simulink model "MIL4L3_SW6_V1_20220211"  (R2018b)
settings: Solver=FixedStepAuto  StartTime=0.0  StopTime=inf  FixedStep=0.001  RelTol=1e-3
PreLoadFcn:
  | A0_MILtest;
undefined symbols (not defined in the file or in its folder): Clb_ICADirect_LaneDisp_StateFive, Clb_ICADirect_LaneDisp_StateFour, Clb_ICADirect_LaneDisp_StateOne, Clb_ICADirect_LaneDisp_StateThree, Clb_ICADirect_LaneDisp_StateTwo, Clb_ICADirect_LaneDisp_StateZero, Clb_ICADirect_LaneDispSW, Clb_ICADirect_TrnLghtsCom_Switch, Clb_ICADirect_TrnLghtsCom_Value, Clb_ICADirect_TrnLghtsCrtl_Inhb, IMAP_Clb_ACU_Driver_Belt, IMAP_Clb_ACU_Driver_Belt_Over, IMAP_Clb_ACU_Passenger_Belt, IMAP_Clb_ACU_Passenger_Belt_Over, IMAP_Clb_ACU_RearLeft_Belt, IMAP_Clb_ACU_RearLeft_Belt_Over, IMAP_Clb_ACU_RearMiddle_Belt, IMAP_Clb_ACU_RearMiddle_Belt_Over, IMAP_Clb_ACU_RearRight_Belt, IMAP_Clb_ACU_RearRight_Belt_Over, IMAP_Clb_AEB_Switch, IMAP_Clb_AEB_Switch_Over, IMAP_Clb_ALC_TLC_Mode, IMAP_Clb_ALC_TLC_Mode_Over, IMAP_Clb_BCM_Battery_Voltage, IMAP_Clb_BCM_Battery_Voltage_Over, IMAP_Clb_BCM_BrakeLamp_State, IMAP_Clb_BCM_BrakeLamp_State_Over, IMAP_Clb_BCM_CHMSL_Status, IMAP_Clb_BCM_CHMSL_Status_Over, IMAP_Clb_BCM_Door_Lock_State, IMAP_Clb_BCM_Door_Lock_State_Over, IMAP_Clb_BCM_FrontWiper_State, IMAP_Clb_BCM_FrontWiper_State_Over, IMAP_Clb_BCM_FrontWiper_Switch, IMAP_Clb_BCM_FrontWiper_Switch_Over, IMAP_Clb_BCM_HazardLamp, IMAP_Clb_BCM_HazardLamp_Over, IMAP_Clb_BCM_HazardLamp_Switch, IMAP_Clb_BCM_HazardLamp_Switch_Over, IMAP_Clb_BCM_HighBeam_State, IMAP_Clb_BCM_HighBeam_State_Over, IMAP_Clb_BCM_Ignition_State, IMAP_Clb_BCM_Ignition_State_Over, IMAP_Clb_BCM_IHBC_Enabled, IMAP_Clb_BCM_IHBC_Enabled_Over, IMAP_Clb_BCM_Left_Light, IMAP_Clb_BCM_Left_Light_Over, IMAP_Clb_BCM_LeftTurn_Switch, IMAP_Clb_BCM_LeftTurn_Switch_Over, IMAP_Clb_BCM_LF_Door_State, IMAP_Clb_BCM_LF_Door_State_Over, IMAP_Clb_BCM_LowBeam_State, IMAP_Clb_BCM_LowBeam_State_Over, IMAP_Clb_BCM_LR_Door_State, IMAP_Clb_BCM_LR_Door_State_Over, IMAP_Clb_BCM_RF_Door_State, IMAP_Clb_BCM_RF_Door_State_Over, IMAP_Clb_BCM_Right_Light, IMAP_Clb_BCM_Right_Light_Over ... (+547)
libraries: CarMaker4SL x2153, simulink x292, dspstat3 x3, canmsglib x2, simulink_extras x1
(part 2 of 52)

== system MIL4L3_SW6_V1_20220211/CarMaker/VehicleControl/OMAP ==
  note: 转向灯控制命令
  note: ACC时距间隔显示
  note: 飞轮扭矩激活请求
  note: 驾驶员设置ACC巡航速度
  note: ACC文字提示
  note: AEB FCW报警请求信号
  note: AEB &FCW Fault 指示灯
  note: AEB OFF指示灯
  note: AEB 文字提示
  note: ACC轮端请求扭矩
  note: ACC状态
  note: 减速度设置
  note: 减速度控制请求
  note: 预建压请求
  note: 减速度类型
  note: AEB状态
  note: 刹车请求(AEB/IBA/ACC共用)
  note: 振动报警请求
  note: 脱手报警
  note: LDW 报警状态
  note: LDW Only 状态指示
  note: 摄像头发出的LKA功能模式
  note: LKA状态指示
  note: LKA功能开启状态
  note: ELK功能指示灯
  note: LKA状态
  note: LKA请求的目标转角
  note: ESA状态
  note: ICA_弹出文字提醒
  note: ICA_状态灯
  note: 多车道模式指示
  note: 提醒驾驶员打转向灯
  note: ESA扭矩请求
  note: ESA请求
  note: 0 No Request
      | 1 左转向灯亮
      | 2 右转向灯亮
      | 3 左右双闪
  note: 1 左
      | 2 右
  Bus Selector2 : BusSelector  Commented=on  OutputSignals=AEBSve_d_Prefill_request,AEBSve_d_functionFARCState,AEBSve_g_DecSetpoint,AEBSve_d_MDDdecRequest,AEBSve_d_MDDdecType,AEBSve_d_ESCDriverOff,AEBSve_d_ESCHoldReq,AEBSve_d_HapticAlarm,AEBSve_d_Braking_progress,AEBSve_d_AEBStatus,AEBSve_d_FCWStatus,AEBSve_d_AEBSwitchStatus,AEBSve_d_AEBFaultStatus,AEBSve_d_AEBAlertReq,AEBSve_d_AEBTips,AEBSve_d_SignalTStamp,AEBSve_d_JABS_AlertSign,AEBSve_d_JABS_SwitchStatus,AEBSve_d_JABS_FltStatus,AEBSve_d_JABS_AlertReq,AEBSve_d_JABS_HapticAlarm,AEBSve_d_JABS_Tips
  Bus Selector3 : BusSelector  OutputSignals=LKASve_y_Vehicle_Lane_Display,LKASve_y_LDW_Status_Display,LKASve_y_LKA_Status_Display,LKASve_y_LDW_Flag,LKASve_y_Hands_Off_Warning,LKASve_y_LKA_Action_Indication,LKASve_y_HMI_Popup_Status,LKASve_y_EPS_State_Control,LKASve_g_LKA_SWA_Control,LKASve_g_EPS_Factor_Control,LKASve_y_EPS_LKA_Control,LKASve_y_LKATorqueReq,LKASve_g_LKATorqueReq_Value
  Bus Selector4 : BusSelector  OutputSignals=JABSve_d_DbPrefillReq,JABSve_d_DbFunFARCSta,JABSve_g_DbDecSetpoint,JABSve_d_DbMDDdecRequest,JABSve_d_DbMDDdecType,JABSve_d_DbHapticAlarm,JABSve_d_DbBraking_progress,JABSve_d_DbSignalTStamp,JABSve_d_DbJACWStatus,JABSve_d_DbSwitchStatus,JABSve_d_DbFltStatus,JABSve_d_DbAlertReq,JABSve_d_DbTips,JABSve_d_DbESCDriveOff,JABSve_d_DbESCHoldReq
  Bus Selector6 : BusSelector  Commented=on  OutputSignals=ELKSve_y_state_ELK_function,ELKSve_y_ELK_HapticAlarmReq,ELKSve_y_Hands_Off_Warning,ELKSve_y_ELK_Action_Indication,ELKSve_y_HMI_Popup_Status,ELKSve_y_EPS_State_Control,ELKSve_g_ELK_SWA_Control,ELKSve_g_EPS_Factor_Control,ELKSve_y_EPS_ELK_Control,ELKSve_y_ELK_VehicleLaneDisp,ELKSve_y_ELK_ELKSts,ELKSve_y_SignalTStamp,ELKSve_y_LKATorqueReq,ELKSve_g_LKATorqueReq_Value
  Bus Selector7 : BusSelector  OutputSignals=IMAPve_d_EPS_LKA_State,IMAPve_g_ESC_LonAcc,IMAPva_d_obj_id,IMAPva_g_obj_pos_x,IMAPve_d_ESC_Veh_Standstill,IMAPve_g_L0_C0,IMAPve_g_L0_C1,IMAPve_g_L0_C2,IMAPve_g_L0_C3,IMAPve_g_R0_C0,IMAPve_g_R0_C1,IMAPve_g_R0_C2,IMAPve_g_R0_C3,IMAPve_d_APA_AutoPark_WorkSt
  Bus Selector8 : BusSelector  Commented=on  OutputSignals=ESASve_y_ESA_State,ESASve_g_ESA_SWA_CMD,ESASve_g_EPS_Factor_Control,ESASve_y_ESA_FaultSt,ESASve_y_ESARequest,ESASve_y_ESATorqueReq,ESASve_y_LKAActivation
  Bus Selector9 : BusSelector  Commented=on  OutputSignals=IMAPve_d_L0_Q,IMAPve_d_R0_Q
  Bus Selector : BusSelector  OutputSignals=FDMMve_d_JaFcnConf,FDMMve_d_AebFcnConf,FDMMve_d_EsaFcnConf,FDMMve_d_ElkFcnConf,FDMMve_d_LkaFcnConf,FDMMve_d_IcaFcnConf,FDMMve_d_AccFcnConf,FDMMve_d_EwFcnConf,FDMMve_g_Adas2Fapa,FDMMve_d_SignalTStamp
  Bus Selector1 : BusSelector  Commented=on  OutputSignals=ACCSve_d_ACC_State,ACCSve_g_ACC_TqReq,ACCSve_d_ACC_TqFlag,ACCSve_g_ACC_DecReq,ACCSve_d_ACC_DecFlag,ACCSve_d_CIPV_ID,ACCSve_d_ACCActive_Signal,ACCSve_d_ACC_go_request,ACCSve_d_VelocitySet,ACCSve_d_HeadWaySet,ACCSve_d_SignalTStamp,ACCSve_d_ACC_ICA_Flag,ACCSve_d_ACC_ESCDriverOff,ACCSve_d_ACC_ESCHoldReq,ACCSve_d_ACC_EPBReq,ACCSve_d_ACCMessagePrompt,ACCSve_d_ACC_ISLCState,ACCSve_d_ACC_ISLCDriverRemind
  Bus Selector5 : BusSelector  Commented=on  OutputSignals=ICABve_d_SignalTStamp,ICABva_d_ICAB2HMI,ICABve_g_SteerAngleCmd,ICABve_d_ICAMode,ICABve_d_ICAState,ICABve_d_LKATorqueReq,ICABve_g_LKATorqueReq_Value
  Data Type  Conversion{,1..2,4..9} (9 alike) : DataTypeConversion
  Data Type Conversion{,2..12,175,180,253..262,264..270,302..304} (34 alike) : DataTypeConversion
  Data Type Conversion1 : DataTypeConversion  Commented=on
  Define CM Dict : CarMaker4SL/Define CM Dict  xname=User.IO.In.ADAS_ACCState  xmono=on  xtype=Int  xdvaplace=None  xnstates=0  xfirststate=0  xinitial=0
  Define CM Dict1 : CarMaker4SL/Define CM Dict  xname=User.IO.In.ADAS_LDWWarningSt  xmono=off  xtype=Double4  xdvaplace=VC  xnstates=0  xfirststate=0  xinitial=0
  Define CM Dict11 : CarMaker4SL/Define CM Dict  xname=User.IO.In.ADAS_LKAAngleReq  xunit=degree  xmono=off  xtype=Double  xdvaplace=IO_In  xnstates=0  xfirststate=0  xinitial=0
  Define CM Dict12 : CarMaker4SL/Define CM Dict  xname=User.IO.In.ADAS_ICAStatusIcon  xmono=off  xtype=Double4  xdvaplace=IO_In  xnstates=0  xfirststate=0  xinitial=0
  Define CM Dict14 : CarMaker4SL/Define CM Dict  xname=User.IO.In.ADAS_ACCTorqueReq  xmono=off  xtype=Double  xdvaplace=None  xnstates=0  xfirststate=0  xinitial=0
  Define CM Dict15 : CarMaker4SL/Define CM Dict  xname=User.IO.In.ADAS_ESCDriveOff  xmono=off  xtype=Double4  xdvaplace=VC  xnstates=0  xfirststate=0  xinitial=0
  Define CM Dict16 : CarMaker4SL/Define CM Dict  xname=User.IO.In.ADAS_ACCSetSpeed  xunit=km/h  xmono=off  xtype=Double  xdvaplace=None  xnstates=0  xfirststate=0  xinitial=0
  Define CM Dict17 : CarMaker4SL/Define CM Dict  xname=User.IO.In.ADAS_ACCHeadwayDisplay  xmono=off  xtype=Double  xdvaplace=None  xnstates=0  xfirststate=0  xinitial=0
  Define CM Dict18 : CarMaker4SL/Define CM Dict  xname=User.IO.In.ADAS_DecelerationSetpoint  xunit=m/s^2  xmono=off  xtype=Double  xdvaplace=None  xnstates=0  xfirststate=0  xinitial=0
  Define CM Dict19 : CarMaker4SL/Define CM Dict  xname=User.IO.In.ADAS_LKAState  xmono=off  xtype=Double  xdvaplace=IO_In  xnstates=0  xfirststate=0  xinitial=0
  Define CM Dict2 : CarMaker4SL/Define CM Dict  Commented=on  xname=User.IO.In.ICA_Mode  xmono=off  xtype=Double4  xdvaplace=VC  xnstates=0  xfirststate=0  xinitial=0
  Define CM Dict20 : CarMaker4SL/Define CM Dict  xname=User.IO.In.ADAS_ISAMessageDisp  xmono=off  xtype=Double4  xdvaplace=IO_In  xnstates=0  xfirststate=0  xinitial=0
  Define CM Dict21 : CarMaker4SL/Define CM Dict  xname=User.IO.In.ADAS_PowerWheelTorqueActiveReq  xmono=off  xtype=Double4  xdvaplace=IO_In  xnstates=0  xfirststate=0  xinitial=0
  Define CM Dict22 : CarMaker4SL/Define CM Dict  xname=User.IO.In.ADAS_ESCHoldReq  xmono=off  xtype=Double4  xdvaplace=VC  xnstates=0  xfirststate=0  xinitial=0
  Define CM Dict23 : CarMaker4SL/Define CM Dict  xname=User.IO.In.ADAS_AEBState  xmono=off  xtype=Double4  xdvaplace=VC  xnstates=0  xfirststate=0  xinitial=0
  Define CM Dict24 : CarMaker4SL/Define CM Dict  xname=User.IO.In.ADAS_AEBAlertReq  xmono=off  xtype=Double4  xdvaplace=VC  xnstates=0  xfirststate=0  xinitial=0
  Define CM Dict25 : CarMaker4SL/Define CM Dict  xname=User.IO.In.ADAS_HapticAlarmRequest  xmono=off  xtype=Double4  xdvaplace=VC  xnstates=0  xfirststate=0  xinitial=0
  Define CM Dict28 : CarMaker4SL/Define CM Dict  xname=User.IO.In.ADAS_DecelerationType  xmono=off  xtype=Double4  xdvaplace=VC  xnstates=0  xfirststate=0  xinitial=0
  Define CM Dict29 : CarMaker4SL/Define CM Dict  xname=User.IO.In.ADAS_DecelerationControlReq  xmono=off  xtype=Double4  xdvaplace=VC  xnstates=0  xfirststate=0  xinitial=0
  Define CM Dict3 : CarMaker4SL/Define CM Dict  xname=User.IO.In.ADAS_ACCMessagePrompt  xmono=off  xtype=Double4  xdvaplace=IO_In  xnstates=0  xfirststate=0  xinitial=0
  Define CM Dict30 : CarMaker4SL/Define CM Dict  xname=User.IO.In.ADAS_AEBFaultStatus  xmono=off  xtype=Double4  xdvaplace=VC  xnstates=0  xfirststate=0  xinitial=0
  Define CM Dict31 : CarMaker4SL/Define CM Dict  xname=User.IO.In.ADAS_AEBSwitchStatus  xmono=off  xtype=Double4  xdvaplace=VC  xnstates=0  xfirststate=0  xinitial=0
  Define CM Dict32 : CarMaker4SL/Define CM Dict  xname=User.IO.In.ADAS_AEBMessageDisp  xmono=off  xtype=Double4  xdvaplace=VC  xnstates=0  xfirststate=0  xinitial=0
  Define CM Dict33 : CarMaker4SL/Define CM Dict  xname=User.IO.In.ADAS_Handoffwarning  xmono=off  xtype=Double4  xdvaplace=VC  xnstates=0  xfirststate=0  xinitial=0
  Define CM Dict34 : CarMaker4SL/Define CM Dict  xname=User.IO.In.ADAS_PrefillRequest  xmono=off  xtype=Double4  xdvaplace=VC  xnstates=0  xfirststate=0  xinitial=0
  Define CM Dict35 : CarMaker4SL/Define CM Dict  xname=User.IO.In.ADAS_ESAFault  xmono=off  xtype=Double4  xdvaplace=IO_In  xnstates=0  xfirststate=0  xinitial=0
  Define CM Dict36 : CarMaker4SL/Define CM Dict  xname=User.IO.In.ADAS_JAFault  xmono=off  xtype=Double4  xdvaplace=IO_In  xnstates=0  xfirststate=0  xinitial=0
  Define CM Dict37 : CarMaker4SL/Define CM Dict  xname=User.IO.In.ADAS_TurnLightsCommand  xmono=off  xtype=Double4  xdvaplace=IO_In  xnstates=0  xfirststate=0  xinitial=0
  Define CM Dict38 : CarMaker4SL/Define CM Dict  xname=User.IO.In.ADAS_ISL_CDriverRemind  xmono=off  xtype=Double  xdvaplace=IO_In  xnstates=0  xfirststate=0  xinitial=0
  Define CM Dict39 : CarMaker4SL/Define CM Dict  xname=User.IO.In.ADAS_LKAStatusDisplay  xmono=off  xtype=Double4  xdvaplace=VC  xnstates=0  xfirststate=0  xinitial=0
  Define CM Dict4 : CarMaker4SL/Define CM Dict  xname=User.IO.In.ADAS_LKASwitchState  xmono=off  xtype=Double4  xdvaplace=VC  xnstates=0  xfirststate=0  xinitial=0
  Define CM Dict40 : CarMaker4SL/Define CM Dict  xname=User.IO.In.ADAS_LKAMode  xmono=off  xtype=Double4  xdvaplace=VC  xnstates=0  xfirststate=0  xinitial=0
  Define CM Dict41 : CarMaker4SL/Define CM Dict  xname=User.IO.In.ADAS_VehicleLaneDisplay  xmono=off  xtype=Double4  xdvaplace=VC  xnstates=0  xfirststate=0  xinitial=0
  Define CM Dict42 : CarMaker4SL/Define CM Dict  xname=User.IO.In.ADAS_HWAActionSts  xmono=off  xtype=Double4  xdvaplace=IO_In  xnstates=0  xfirststate=0  xinitial=0
  Define CM Dict44 : CarMaker4SL/Define CM Dict  xname=User.IO.In.ADAS_LDWStatusDisplay  xmono=off  xtype=Double4  xdvaplace=VC  xnstates=0  xfirststate=0  xinitial=0
  Define CM Dict48 : CarMaker4SL/Define CM Dict  xname=User.IO.In.ADAS_HWAMode  xmono=off  xtype=Double4  xdvaplace=IO_In  xnstates=0  xfirststate=0  xinitial=0
  Define CM Dict5 : CarMaker4SL/Define CM Dict  xname=User.IO.In.ADAS_ELKSts  xmono=off  xtype=Double4  xdvaplace=VC  xnstates=0  xfirststate=0  xinitial=0
  Define CM Dict50 : CarMaker4SL/Define CM Dict  xname=User.IO.In.ADAS_HWATurnOnIndicator  xmono=off  xtype=Double4  xdvaplace=IO_In  xnstates=0  xfirststate=0  xinitial=0
  Define CM Dict51 : CarMaker4SL/Define CM Dict  xname=User.IO.In.ADAS_ESATorqueReq  xmono=off  xtype=Double  xdvaplace=IO_In  xnstates=0  xfirststate=0  xinitial=0
  Define CM Dict52 : CarMaker4SL/Define CM Dict  xname=User.IO.In.ADAS_ESARequest  xmono=off  xtype=Double  xdvaplace=IO_In  xnstates=0  xfirststate=0  xinitial=0
  Define CM Dict6 : CarMaker4SL/Define CM Dict  xname=User.IO.In.ADAS_ESAState  xmono=off  xtype=Double  xdvaplace=IO_In  xnstates=0  xfirststate=0  xinitial=0
  Define CM Dict7 : CarMaker4SL/Define CM Dict  xname=User.IO.In.ADAS_ISLCState  xmono=off  xtype=Double  xdvaplace=IO_In  xnstates=0  xfirststate=0  xinitial=0
  Define CM Dict8 : CarMaker4SL/Define CM Dict  xname=User.IO.In.ADAS_ACCHeadwayIcon  xmono=off  xtype=Double  xdvaplace=None  xnstates=0  xfirststate=0  xinitial=0
  Define CM Dict9 : CarMaker4SL/Define CM Dict  xname=User.IO.In.ADAS_BrakeRequest  xmono=off  xtype=Double4  xdvaplace=VC  xnstates=0  xfirststate=0  xinitial=0
  Delay : Delay  DelayLength=1
  From : From  Commented=on  GotoTag=ESA_output  TagVisibility=global
  From19 : From  Commented=on  GotoTag=ACC_output  TagVisibility=global
  From33 : From  Commented=on  GotoTag=AEB_output  TagVisibility=global
  From37 : From  Commented=on  GotoTag=ELK_output  TagVisibility=global
  From38 : From  Commented=on  GotoTag=ICAB_output  TagVisibility=global
  Goto7 : Goto  Commented=on  GotoTag=Decel_Request  TagVisibility=global
  Manual Switch : ManualSwitch
  OMAP1 : Subsystem  TreatAsAtomicUnit=on  SystemSampleTime=0.01
  Write CM Dict : CarMaker4SL/Write CM Dict  xname=User.IO.In.ADAS_LDWWarningSt  xsync=off
  Write CM Dict1 : CarMaker4SL/Write CM Dict  xname=User.IO.In.ADAS_BrakeRequest  xsync=off
  Write CM Dict10 : CarMaker4SL/Write CM Dict  xname=User.IO.In.ADAS_ISAMessageDisp  xsync=off
  Write CM Dict11 : CarMaker4SL/Write CM Dict  xname=User.IO.In.ADAS_LKAState  xsync=off
  Write CM Dict12 : CarMaker4SL/Write CM Dict  xname=User.IO.In.ADAS_PowerWheelTorqueActiveReq  xsync=off
  Write CM Dict13 : CarMaker4SL/Write CM Dict  xname=User.IO.In.ADAS_ACCMessagePrompt  xsync=off
  Write CM Dict14 : CarMaker4SL/Write CM Dict  xname=User.IO.In.ADAS_AEBState  xsync=off
  Write CM Dict15 : CarMaker4SL/Write CM Dict  xname=User.IO.In.ADAS_AEBAlertReq  xsync=off
  Write CM Dict16 : CarMaker4SL/Write CM Dict  xname=User.IO.In.ADAS_HapticAlarmRequest  xsync=off
  Write CM Dict19 : CarMaker4SL/Write CM Dict  xname=User.IO.In.ADAS_DecelerationType  xsync=off
  Write CM Dict2 : CarMaker4SL/Write CM Dict  xname=User.IO.In.ADAS_ACCState  xsync=off
  Write CM Dict20 : CarMaker4SL/Write CM Dict  xname=User.IO.In.ADAS_DecelerationControlReq  xsync=off
  Write CM Dict21 : CarMaker4SL/Write CM Dict  xname=User.IO.In.ADAS_AEBFaultStatus  xsync=off
  Write CM Dict22 : CarMaker4SL/Write CM Dict  xname=User.IO.In.ADAS_AEBSwitchStatus  xsync=off
  Write CM Dict23 : CarMaker4SL/Write CM Dict  xname=User.IO.In.ADAS_AEBMessageDisp  xsync=off
  Write CM Dict24 : CarMaker4SL/Write CM Dict  xname=User.IO.In.ADAS_Handoffwarning  xsync=off
  Write CM Dict25 : CarMaker4SL/Write CM Dict  xname=User.IO.In.ADAS_PrefillRequest  xsync=off
  Write CM Dict26 : CarMaker4SL/Write CM Dict  Commented=on  xname=User.IO.In.ICA_Mode  xsync=off
  Write CM Dict27 : CarMaker4SL/Write CM Dict  xname=User.IO.In.ADAS_LKAStatusDisplay  xsync=off
  Write CM Dict28 : CarMaker4SL/Write CM Dict  xname=User.IO.In.ADAS_LKAMode  xsync=off
  Write CM Dict29 : CarMaker4SL/Write CM Dict  xname=User.IO.In.ADAS_LDWStatusDisplay  xsync=off
  Write CM Dict30 : CarMaker4SL/Write CM Dict  xname=User.IO.In.ADAS_HWAMode  xsync=off
  Write CM Dict31 : CarMaker4SL/Write CM Dict  xname=User.IO.In.ADAS_LKASwitchState  xsync=off
  Write CM Dict32 : CarMaker4SL/Write CM Dict  xname=User.IO.In.ADAS_ELKSts  xsync=off
  Write CM Dict33 : CarMaker4SL/Write CM Dict  xname=User.IO.In.ADAS_ESAState  xsync=off
  Write CM Dict34 : CarMaker4SL/Write CM Dict  xname=User.IO.In.ADAS_HWATurnOnIndicator  xsync=off
  Write CM Dict35 : CarMaker4SL/Write CM Dict  xname=User.IO.In.ADAS_ESATorqueReq  xsync=off
  Write CM Dict36 : CarMaker4SL/Write CM Dict  xname=User.IO.In.ADAS_ESARequest  xsync=off
  Write CM Dict37 : CarMaker4SL/Write CM Dict  xname=User.IO.In.ADAS_ISLCState  xsync=off
  Write CM Dict38 : CarMaker4SL/Write CM Dict  xname=User.IO.In.ADAS_ACCHeadwayIcon  xsync=off
  Write CM Dict39 : CarMaker4SL/Write CM Dict  xname=User.IO.In.ADAS_ESCDriveOff  xsync=off
  Write CM Dict4 : CarMaker4SL/Write CM Dict  xname=User.IO.In.ADAS_ACCTorqueReq  xsync=off
  Write CM Dict40 : CarMaker4SL/Write CM Dict  xname=User.IO.In.ADAS_ESCHoldReq  xsync=off
  Write CM Dict41 : CarMaker4SL/Write CM Dict  xname=User.IO.In.ADAS_ESAFault  xsync=off
  Write CM Dict42 : CarMaker4SL/Write CM Dict  xname=User.IO.In.ADAS_JAFault  xsync=off
  Write CM Dict43 : CarMaker4SL/Write CM Dict  xname=User.IO.In.ADAS_TurnLightsCommand  xsync=off
  Write CM Dict44 : CarMaker4SL/Write CM Dict  xname=User.IO.In.ADAS_ISL_CDriverRemind  xsync=off
  Write CM Dict45 : CarMaker4SL/Write CM Dict  xname=User.IO.In.ADAS_VehicleLaneDisplay  xsync=off
  Write CM Dict46 : CarMaker4SL/Write CM Dict  xname=User.IO.In.ADAS_HWAActionSts  xsync=off
  Write CM Dict5 : CarMaker4SL/Write CM Dict  xname=User.IO.In.ADAS_ACCSetSpeed  xsync=off
  Write CM Dict6 : CarMaker4SL/Write CM Dict  xname=User.IO.In.ADAS_ACCHeadwayDisplay  xsync=off
  Write CM Dict7 : CarMaker4SL/Write CM Dict  xname=User.IO.In.ADAS_DecelerationSetpoint  xsync=off
  Write CM Dict8 : CarMaker4SL/Write CM Dict  xname=User.IO.In.ADAS_LKAAngleReq  xsync=off
  Write CM Dict9 : CarMaker4SL/Write CM Dict  xname=User.IO.In.ADAS_ICAStatusIcon  xsync=off
  tag scope: ACCTqReq=global, ADAS_AEBAlertReq=global, ADAS_DecelerationSet=global, ADAS_TorqueActivReq=global, MDD_Decelerationcontrol_request=global, MDD_deceleration_type=global
  wires:
  [JA_output] -> Bus Selector4/1
  From33/1 -> Bus Selector2/1
  From19/1 -> Bus Selector1/1
  [LKA_output] -> Bus Selector3/1
  From38/1 -> Bus Selector5/1
  [FDMM_output] -> Bus Selector/1
  Data Type Conversion302/1 -> Write CM Dict27/1
  From37/1 -> Bus Selector6/1
  Data Type Conversion260/1 -> Write CM Dict13/1
  Data Type Conversion264/1 -> Write CM Dict19/1
  Data Type Conversion1/1 -> Write CM Dict26/1
  Data Type Conversion304/1 -> Write CM Dict29/1
  Data Type Conversion268/1 -> Write CM Dict23/1
  Data Type  Conversion1/1 -> Write CM Dict10/1
  Data Type Conversion259/1 -> Write CM Dict12/1
  Data Type Conversion267/1 -> Write CM Dict22/1
  Data Type Conversion253/1 -> Write CM Dict5/1
  Data Type Conversion258/1 -> Write CM Dict11/1
  Data Type Conversion303/1 -> Write CM Dict28/1
  Data Type Conversion/1 -> Write CM Dict2/1
  Data Type Conversion175/1 -> Write CM Dict/1
  OMAP1/10(OMAPve_y_ADAS_AEBAlertReq) -> Data Type Conversion261/1, [ADAS_AEBAlertReq]
  Manual Switch/1 -> Data Type  Conversion/1
  Data Type Conversion257/1 -> Write CM Dict8/1
  Data Type  Conversion/1 -> Write CM Dict9/1
  Data Type Conversion262/1 -> Write CM Dict16/1
  Data Type Conversion270/1 -> Write CM Dict25/1
  Data Type Conversion266/1 -> Write CM Dict21/1
  Bus Selector5/4 -> OMAP1/96(ICABve_d_ICAMode), Data Type Conversion1/1  "<ICABve_d_ICAMode>"
  Data Type Conversion269/1 -> Write CM Dict24/1
  Data Type Conversion265/1 -> Write CM Dict20/1
  Data Type Conversion254/1 -> Write CM Dict6/1
  Data Type Conversion256/1 -> Write CM Dict4/1
  Data Type  Conversion2/1 -> Write CM Dict14/1
  Data Type Conversion255/1 -> Write CM Dict7/1
  Data Type Conversion180/1 -> Write CM Dict1/1
  Data Type Conversion2/1 -> Write CM Dict31/1
  Data Type Conversion3/1 -> Write CM Dict32/1
  Data Type Conversion4/1 -> Write CM Dict33/1
  Bus Selector2/1 -> OMAP1/29(AEBSve_d_Prefill_request)  "<AEBSve_d_Prefill_request>"
  Bus Selector2/2 -> OMAP1/30(AEBSve_d_functionFARCState)  "<AEBSve_d_functionFARCState>"
  Bus Selector2/3 -> OMAP1/31(AEBSve_g_DecSetpoint)  "<AEBSve_g_DecSetpoint>"
  Bus Selector2/4 -> OMAP1/32(AEBSve_d_MDDdecRequest)  "<AEBSve_d_MDDdecRequest>"
  Bus Selector2/5 -> OMAP1/33(AEBSve_d_MDDdecType)  "<AEBSve_d_MDDdecType>"
  Bus Selector2/6 -> OMAP1/34(AEBSve_d_ESCDriveOff)  "<AEBSve_d_ESCDriverOff>"
  Bus Selector2/7 -> OMAP1/35(AEBSve_d_ESCHoldReq)  "<AEBSve_d_ESCHoldReq>"
  Bus Selector2/8 -> OMAP1/36(AEBSve_d_HapticAlarm)  "<AEBSve_d_HapticAlarm>"
  Bus Selector2/9 -> OMAP1/37(AEBSve_d_Braking_progress)  "<AEBSve_d_Braking_progress>"
  Bus Selector2/10 -> OMAP1/38(AEBSve_d_AEBStatus)  "<AEBSve_d_AEBStatus>"
  Bus Selector2/11 -> OMAP1/39(AEBSve_d_FCWStatus)  "<AEBSve_d_FCWStatus>"
  Bus Selector2/12 -> OMAP1/40(AEBSve_d_AEBSwitchStatus)  "<AEBSve_d_AEBSwitchStatus>"
  Bus Selector2/13 -> OMAP1/41(AEBSve_d_AEBFaultStatus)  "<AEBSve_d_AEBFaultStatus>"
  Bus Selector2/14 -> OMAP1/42(AEBSve_d_AEBAlertReq)  "<AEBSve_d_AEBAlertReq>"
  Bus Selector2/15 -> OMAP1/43(AEBSve_d_AEBTips)  "<AEBSve_d_AEBTips>"
  Bus Selector2/16 -> OMAP1/44(AEBSve_d_SignalTStamp)  "<AEBSve_d_SignalTStamp>"
  Bus Selector2/17 -> OMAP1/45(AEBSve_d_JABS_AlertSign)  "<AEBSve_d_JABS_AlertSign>"
  Bus Selector2/18 -> OMAP1/46(AEBSve_d_JABS_SwitchStatus)  "<AEBSve_d_JABS_SwitchStatus>"
  Bus Selector2/19 -> OMAP1/47(AEBSve_d_JABS_FltStatus)  "<AEBSve_d_JABS_FltStatus>"
  Bus Selector2/20 -> OMAP1/48(AEBSve_d_JABS_AlertReq)  "<AEBSve_d_JABS_AlertReq>"
  Bus Selector2/21 -> OMAP1/49(AEBSve_d_JABS_HapticAlarm)  "<AEBSve_d_JABS_HapticAlarm>"
  Bus Selector2/22 -> OMAP1/50(AEBSve_d_JABS_Tips)  "<AEBSve_d_JABS_Tips>"
  Bus Selector4/1 -> OMAP1/51(JABSve_d_DbPrefillReq)  "<JABSve_d_DbPrefillReq>"
  Bus Selector4/2 -> OMAP1/52(JABSve_d_DbFunFARCSta)  "<JABSve_d_DbFunFARCSta>"
  Bus Selector4/3 -> OMAP1/53(JABSve_g_DbDecSetpoint)  "<JABSve_g_DbDecSetpoint>"
  Bus Selector4/4 -> OMAP1/54(JABSve_d_DbMDDdecRequest)  "<JABSve_d_DbMDDdecRequest>"
  Bus Selector4/5 -> OMAP1/55(JABSve_d_DbMDDdecType)  "<JABSve_d_DbMDDdecType>"
  Bus Selector4/6 -> OMAP1/56(JABSve_d_DbHapticAlarm)  "<JABSve_d_DbHapticAlarm>"
  Bus Selector4/7 -> OMAP1/57(JABSve_d_DbBraking_progress)  "<JABSve_d_DbBraking_progress>"
  Bus Selector4/8 -> OMAP1/58(JABSve_d_DbSignalTStamp)  "<JABSve_d_DbSignalTStamp>"
  Bus Selector5/3 -> OMAP1/95(ICABve_g_SteerAngleCmd)  "<ICABve_g_SteerAngleCmd>"
  OMAP1/3(OMAPve_y_ADAS_ACCHeadwayDisplay) -> Data Type Conversion254/1
  OMAP1/5(OMAPve_y_ADAS_ACCSetSpeed) -> Data Type Conversion253/1
  OMAP1/9(OMAPve_y_ADAS_ACCMessagePrompt) -> Data Type Conversion260/1
  OMAP1/11(OMAPve_y_ADAS_AEBFaultStatus) -> Data Type Conversion266/1
  OMAP1/13(OMAPve_y_ADAS_AEBMassageDisp) -> Data Type Conversion268/1
  OMAP1/14(OMAPve_g_ADAS_ACCTorqueReq) -> [ACCTqReq], Data Type Conversion256/1
  OMAP1/15(OMAPve_y_ADAS_TorqueActivReq) -> [ADAS_TorqueActivReq], Data Type Conversion259/1
  OMAP1/18(OMAPve_y_ADAS_ACCState) -> Data Type Conversion/1
  OMAP1/19(OMAPve_g_ADAS_DecelerationSet) -> Data Type Conversion255/1, [ADAS_DecelerationSet]
  OMAP1/20(OMAPve_y_ADAS_DeclControlReq) -> Data Type Conversion265/1, [MDD_Decelerationcontrol_request]
  OMAP1/21(OMAPve_y_ADAS_PrefillRequest) -> Data Type Conversion270/1
  OMAP1/24(OMAPve_y_ADAS_DecelerationType) -> Data Type Conversion264/1, Delay/1
  OMAP1/25(OMAPve_y_ADAS_AEBState) -> Data Type  Conversion2/1
  OMAP1/26(OMAPve_y_ADAS_BrakeRequest) -> Goto7/1, Data Type Conversion180/1
  OMAP1/28(OMAPve_y_ADAS_HapticAlarmReq) -> Data Type Conversion262/1
  OMAP1/29(OMAPve_y_ADAS_Handsoffwarning) -> Data Type Conversion269/1
  OMAP1/37(OMAPve_y_ADAS_ELKSts) -> Data Type Conversion3/1
  OMAP1/36(OMAPve_y_ADAS_LKASwitchState) -> Data Type Conversion2/1
  OMAP1/35(OMAPve_y_ADAS_LKAStatusDisplay) -> Data Type Conversion302/1
  OMAP1/34(OMAPve_y_ADAS_LKAMode) -> Data Type Conversion303/1
  OMAP1/33(OMAPve_y_ADAS_LDWStatusDisplay) -> Data Type Conversion304/1
  OMAP1/32(OMAPve_y_ADAS_LDWWarningSt) -> Data Type Conversion175/1
  OMAP1/40(OMAPve_y_ADAS_LKAState) -> Data Type Conversion258/1
  OMAP1/44(OMAPve_y_ADAS_ESAState) -> Data Type Conversion4/1
  OMAP1/47(OMAPve_y_ADAS_ICAMassageDisp) -> Data Type  Conversion1/1
  OMAP1/48(OMAPve_y_ADAS_ICAStatusIcon) -> Manual Switch/1
  [ICABve_d_ICAState] -> Manual Switch/2
  Bus Selector3/1 -> OMAP1/66(LKASve_y_Vehicle_Lane_Display)  "<LKASve_y_Vehicle_Lane_Display>"
  Bus Selector3/2 -> OMAP1/67(LKASve_y_LDW_Status_Display)  "<LKASve_y_LDW_Status_Display>"
  Bus Selector3/3 -> OMAP1/68(LKASve_y_LKA_Status_Display)  "<LKASve_y_LKA_Status_Display>"
  Bus Selector3/4 -> OMAP1/69(LKASve_y_LDW_Flag)  "<LKASve_y_LDW_Flag>"
  Bus Selector3/5 -> OMAP1/70(LKASve_y_Hands_Off_Warning)  "<LKASve_y_Hands_Off_Warning>"
  Bus Selector3/6 -> OMAP1/71(LKASve_y_LKA_Action_Indication)  "<LKASve_y_LKA_Action_Indication>"
  Bus Selector3/7 -> OMAP1/72(LKASve_y_HMI_Popup_Status)  "<LKASve_y_HMI_Popup_Status>"
  Bus Selector3/8 -> OMAP1/73(LKASve_y_EPS_State_Control)  "<LKASve_y_EPS_State_Control>"
  Bus Selector3/9 -> OMAP1/74(LKASve_g_LKA_SWA_Control)  "<LKASve_g_LKA_SWA_Control>"
  Bus Selector3/10 -> OMAP1/75(LKASve_g_EPS_Factor_Control)  "<LKASve_g_EPS_Factor_Control>"
  Bus Selector3/11 -> OMAP1/76(LKASve_y_EPS_LKA_Control)  "<LKASve_y_EPS_LKA_Control>"
  Bus Selector3/12 -> OMAP1/77(LKASve_y_LKATorqueReq)  "<LKASve_y_LKATorqueReq>"
  Bus Selector3/13 -> OMAP1/78(LKASve_g_LKATorqueReq_Value)  "<LKASve_g_LKATorqueReq_Value>"
  Delay/1 -> [MDD_deceleration_type]
  Bus Selector4/9 -> OMAP1/59(JABSve_d_DbJACWStatus)  "<JABSve_d_DbJACWStatus>"
  Bus Selector4/10 -> OMAP1/60(JABSve_d_DbSwitchStatus)  "<JABSve_d_DbSwitchStatus>"
  Bus Selector4/11 -> OMAP1/61(JABSve_d_DbFltStatus)  "<JABSve_d_DbFltStatus>"
  Bus Selector4/12 -> OMAP1/62(JABSve_d_DbAlertReq)  "<JABSve_d_DbAlertReq>"
  Bus Selector4/13 -> OMAP1/63(JABSve_d_DbTips)  "<JABSve_d_DbTips>"
  Bus Selector4/14 -> OMAP1/64(JABSve_d_DbESCDriveOff)  "<JABSve_d_DbESCDriveOff>"
  Bus Selector4/15 -> OMAP1/65(JABSve_d_DbESCHoldReq)  "<JABSve_d_DbESCHoldReq>"
  Bus Selector6/1 -> OMAP1/79(ELKSve_y_state_ELK_function)  "<ELKSve_y_state_ELK_function>"
  Bus Selector6/2 -> OMAP1/80(ELKSve_y_ELK_HapticAlarmReq)  "<ELKSve_y_ELK_HapticAlarmReq>"
  Bus Selector6/3 -> OMAP1/81(ELKSve_y_Hands_Off_Warning)  "<ELKSve_y_Hands_Off_Warning>"
  Bus Selector6/4 -> OMAP1/82(ELKSve_y_ELK_Action_Indication)  "<ELKSve_y_ELK_Action_Indication>"
  Bus Selector6/5 -> OMAP1/83(ELKSve_y_HMI_Popup_Status)  "<ELKSve_y_HMI_Popup_Status>"
  Bus Selector6/6 -> OMAP1/84(ELKSve_y_EPS_State_Control)  "<ELKSve_y_EPS_State_Control>"
  Bus Selector6/7 -> OMAP1/85(ELKSve_g_ELK_SWA_Control)  "<ELKSve_g_ELK_SWA_Control>"
  Bus Selector6/8 -> OMAP1/86(ELKSve_g_EPS_Factor_Control)  "<ELKSve_g_EPS_Factor_Control>"
  Bus Selector6/9 -> OMAP1/87(ELKSve_y_EPS_ELK_Control)  "<ELKSve_y_EPS_ELK_Control>"
  Bus Selector6/10 -> OMAP1/88(ELKSve_y_ELK_VehicleLaneDisp)  "<ELKSve_y_ELK_VehicleLaneDisp>"
  Bus Selector6/11 -> OMAP1/89(ELKSve_y_ELK_ELKSts)  "<ELKSve_y_ELK_ELKSts>"
  Bus Selector6/12 -> OMAP1/90(ELKSve_y_SignalTStamp)  "<ELKSve_y_SignalTStamp>"
  Bus Selector6/13 -> OMAP1/91(ELKSve_y_LKATorqueReq)  "<ELKSve_y_LKATorqueReq>"
  Bus Selector6/14 -> OMAP1/92(ELKSve_g_LKATorqueReq_Value)  "<ELKSve_g_LKATorqueReq_Value>"
  OMAP1/49(OMAPve_y_ADAS_HWAMode) -> Data Type  Conversion4/1
  Data Type  Conversion4/1 -> Write CM Dict30/1
  OMAP1/50(OMAPve_y_ADAS_HWATurnOnIdctr) -> Data Type  Conversion5/1
  Data Type  Conversion5/1 -> Write CM Dict34/1  "ADAS_HWATurnOnIndicator"
  OMAP1/45(OMAPve_g_ADAS_ESATorqueReq) -> Data Type Conversion5/1
  Data Type Conversion5/1 -> Write CM Dict35/1
  OMAP1/46(OMAPve_y_ADAS_ESARequest) -> Data Type Conversion6/1
  Data Type Conversion6/1 -> Write CM Dict36/1
  ? -> ?
  Bus Selector/1 -> OMAP1/1(FDMMve_d_JaFcnConf)  "<FDMMve_d_JaFcnConf>"
  Bus Selector/2 -> OMAP1/2(FDMMve_d_AebFcnConf)  "<FDMMve_d_AebFcnConf>"
  Bus Selector/3 -> OMAP1/3(FDMMve_d_EsaFcnConf)  "<FDMMve_d_EsaFcnConf>"
  Bus Selector/4 -> OMAP1/4(FDMMve_d_ElkFcnConf)  "<FDMMve_d_ElkFcnConf>"
  Bus Selector/5 -> OMAP1/5(FDMMve_d_LkaFcnConf)  "<FDMMve_d_LkaFcnConf>"
  Bus Selector/6 -> OMAP1/6(FDMMve_d_IcaFcnConf)  "<FDMMve_d_IcaFcnConf>"
  Bus Selector/7 -> OMAP1/7(FDMMve_d_AccFcnConf)  "<FDMMve_d_AccFcnConf>"
  Bus Selector/8 -> OMAP1/8(FDMMve_d_EwFcnConf)  "<FDMMve_d_EwFcnConf>"
  Bus Selector/9 -> OMAP1/9(FDMMve_g_Adas2Fapa)  "<FDMMve_g_Adas2Fapa>"
  Bus Selector/10 -> OMAP1/10(FDMMve_d_SignalTStamp)  "<FDMMve_d_SignalTStamp>"
  Bus Selector1/1 -> OMAP1/11(ACCSve_d_ACC_State)  "<ACCSve_d_ACC_State>"
  Bus Selector1/2 -> OMAP1/12(ACCSve_g_ACC_TqReq)  "<ACCSve_g_ACC_TqReq>"
  Bus Selector1/3 -> OMAP1/13(ACCSve_d_ACC_TqFlag)  "<ACCSve_d_ACC_TqFlag>"
  Bus Selector1/4 -> OMAP1/14(ACCSve_g_ACC_DecReq)  "<ACCSve_g_ACC_DecReq>"
  Bus Selector1/5 -> OMAP1/15(ACCSve_d_ACC_DecFlag)  "<ACCSve_d_ACC_DecFlag>"
  Bus Selector1/6 -> OMAP1/16(ACCSve_d_CIPV_ID)  "<ACCSve_d_CIPV_ID>"
  Bus Selector1/7 -> OMAP1/17(ACCSve_d_ACCActive_Signal)  "<ACCSve_d_ACCActive_Signal>"
  Bus Selector1/8 -> OMAP1/18(ACCSve_d_ACC_go_request)  "<ACCSve_d_ACC_go_request>"
  Bus Selector1/9 -> OMAP1/19(ACCSve_d_VelocitySet)  "<ACCSve_d_VelocitySet>"
  Bus Selector1/10 -> OMAP1/20(ACCSve_d_HeadWaySet)  "<ACCSve_d_HeadWaySet>"
  Bus Selector1/11 -> OMAP1/21(ACCSve_d_SignalTStamp)  "<ACCSve_d_SignalTStamp>"
  Bus Selector1/12 -> OMAP1/22(ACCSve_d_ACC_ICA_Flag)  "<ACCSve_d_ACC_ICA_Flag>"
  Bus Selector1/13 -> OMAP1/23(ACCSve_d_ACC_ESCDriveOff)  "<ACCSve_d_ACC_ESCDriverOff>"
  Bus Selector1/14 -> OMAP1/24(ACCSve_d_ACC_ESCHoldReq)  "<ACCSve_d_ACC_ESCHoldReq>"
  Bus Selector1/15 -> OMAP1/25(ACCSve_d_ACC_EPBReq)  "<ACCSve_d_ACC_EPBReq>"
  Bus Selector1/16 -> OMAP1/26(ACCSve_d_ACCMessagePrompt)  "<ACCSve_d_ACCMessagePrompt>"
  Bus Selector1/17 -> OMAP1/27(ACCSve_d_ACC_ISLCState)  "<ACCSve_d_ACC_ISLCState>"
  Bus Selector1/18 -> OMAP1/28(ACCSve_d_ACC_ISLCDriverRemind)  "<ACCSve_d_ACC_ISLCDriverRemind>"
  [IMAP_Output] -> Bus Selector9/1, Bus Selector7/1
  OMAP1/12(OMAPve_y_ADAS_AEBSwitchStatus) -> Data Type Conversion267/1
  OMAP1/1(OMAPve_y_ADAS_ISLCState) -> Data Type Conversion7/1
  Data Type Conversion7/1 -> Write CM Dict37/1
  OMAP1/4(OMAPve_y_ADAS_ACCHeadwayIcon) -> Data Type Conversion8/1
  Data Type Conversion8/1 -> Write CM Dict38/1
  OMAP1/22(OMAPve_y_ADAS_ESCDriveOff) -> Data Type Conversion9/1
  Data Type Conversion9/1 -> Write CM Dict39/1
  Data Type Conversion10/1 -> Write CM Dict40/1
  OMAP1/23(OMAPve_y_ADAS_ESCHoldReq) -> Data Type Conversion10/1
  Data Type  Conversion6/1 -> Write CM Dict41/1
  OMAP1/51(OMAPve_y_ADAS_ESAFaultSt) -> Data Type  Conversion6/1
  OMAP1/52(OMAPve_y_ADAS_JAFaultSt) -> Data Type  Conversion7/1
  Data Type  Conversion7/1 -> Write CM Dict42/1
  OMAP1/59(OMAPve_y_ADAS_TurnLightsCommand) -> Data Type  Conversion8/1
  Data Type  Conversion8/1 -> Write CM Dict43/1
  Bus Selector5/6 -> OMAP1/98(ICABve_d_LKATorqueReq)  "<ICABve_d_LKATorqueReq>"
  Bus Selector5/1 -> OMAP1/93(ICABve_d_SignalTStamp)  "<ICABve_d_SignalTStamp>"
  Bus Selector5/2 -> OMAP1/94(ICABva_d_ICAB2HMI)  "<ICABva_d_ICAB2HMI>"
  Data Type Conversion11/1 -> Write CM Dict44/1
  OMAP1/2(OMAPve_y_ADAS_ISLCDriverRemind) -> Data Type Conversion11/1
  OMAP1/31(OMAPve_y_ADAS_VehicleLaneDisp) -> Data Type Conversion12/1
  Data Type Conversion12/1 -> Write CM Dict45/1
  From/1 -> Bus Selector8/1
  Bus Selector8/3 -> OMAP1/116(ESASve_g_EPS_Factor_Control)  "<ESASve_g_EPS_Factor_Control>"
  Bus Selector8/2 -> OMAP1/115(ESASve_g_ESA_SWA_CMD)  "<ESASve_g_ESA_SWA_CMD>"
  Bus Selector8/4 -> OMAP1/117(ESASve_y_ESA_FaultSt)  "<ESASve_y_ESA_FaultSt>"
  Bus Selector8/1 -> OMAP1/114(ESASve_y_ESA_State)  "<ESASve_y_ESA_State>"
  Bus Selector8/5 -> OMAP1/118(ESASve_y_ESARequest)  "<ESASve_y_ESARequest>"
  Bus Selector8/6 -> OMAP1/119(ESASve_y_ESATorqueReq)  "<ESASve_y_ESATorqueReq>"
  Bus Selector8/7 -> OMAP1/120(ESASve_y_LKAActivation)  "<ESASve_y_LKAActivation>"
  OMAP1/53(OMAPve_y_ADAS_HWAActionSts) -> Data Type  Conversion9/1
  Data Type  Conversion9/1 -> Write CM Dict46/1
  Bus Selector5/5 -> OMAP1/97(ICABve_d_ICAState)  "<ICABve_d_ICAState>"
  Bus Selector5/7 -> OMAP1/99(ICABve_g_LKATorqueReq_Value)  "<ICABve_g_LKATorqueReq_Value>"
  Bus Selector7/1 -> OMAP1/100(IMAPve_d_EPS_LKA_State)  "<IMAPve_d_EPS_LKA_State>"
  Bus Selector7/2 -> OMAP1/101(IMAPve_g_ESC_LonAcc)  "<IMAPve_g_ESC_LonAcc>"
  Bus Selector7/3 -> OMAP1/102(IMAPva_d_obj_id)  "<IMAPva_d_obj_id>"
  Bus Selector7/4 -> OMAP1/103(IMAPva_g_obj_pos_x)  "<IMAPva_g_obj_pos_x>"
  Bus Selector7/5 -> OMAP1/104(IMAPve_d_ESC_Veh_Standstill)  "<IMAPve_d_ESC_Veh_Standstill>"
  Bus Selector7/6 -> OMAP1/105(IMAPve_g_L0_C0)  "<IMAPve_g_L0_C0>"
  Bus Selector7/7 -> OMAP1/106(IMAPve_g_L0_C1)  "<IMAPve_g_L0_C1>"
  Bus Selector7/11 -> OMAP1/110(IMAPve_g_R0_C1)  "<IMAPve_g_R0_C1>"
  Bus Selector7/12 -> OMAP1/111(IMAPve_g_R0_C2)  "<IMAPve_g_R0_C2>"
  Bus Selector7/13 -> OMAP1/112(IMAPve_g_R0_C3)  "<IMAPve_g_R0_C3>"
  Bus Selector7/14 -> OMAP1/113(IMAPve_d_APA_AutoPark_WorkSt)  "<IMAPve_d_APA_AutoPark_WorkSt>"
  OMAP1/42(OMAPve_g_ADAS_LKAAngleReq) -> Data Type Conversion257/1
  Bus Selector9/1 -> OMAP1/121(IMAPve_d_L0_Q)  "<IMAPve_d_L0_Q>"
  Bus Selector9/2 -> OMAP1/122(IMAPve_d_R0_Q)  "<IMAPve_d_R0_Q>"
  Bus Selector7/8 -> OMAP1/107(IMAPve_g_L0_C2)  "<IMAPve_g_L0_C2>"
  Bus Selector7/9 -> OMAP1/108(IMAPve_g_L0_C3)  "<IMAPve_g_L0_C3>"
  Bus Selector7/10 -> OMAP1/109(IMAPve_g_R0_C0)  "<IMAPve_g_R0_C0>"
  Data Type Conversion261/1 -> Write CM Dict15/1

== system MIL4L3_SW6_V1_20220211/CarMaker/VehicleControl/PowerControl ==
  AM_PwrSupCurrentMor : Subsystem
  AM_PwrSupVoltageMor : Subsystem
  Constant : Constant  Value=0
  Define CM Dict1 : CarMaker4SL/Define CM Dict  xname=User.IO.Out.PwrSupUctrl  xmono=off  xtype=Double4  xdvaplace=IO_Out  xnstates=0  xfirststate=0  xinitial=0
  Define CM Dict2 : CarMaker4SL/Define CM Dict  xname=User.IO.Out.PwrSupUctrl_SW  xmono=off  xtype=Double4  xdvaplace=IO_Out  xnstates=0  xfirststate=0  xinitial=0
  Define CM Dict41 : CarMaker4SL/Define CM Dict  xname=User.IO.Out.KL30  xmono=off  xtype=Double4  xdvaplace=IO_Out  xnstates=0  xfirststate=0  xinitial=0
  Define CM Dict42 : CarMaker4SL/Define CM Dict  xname=User.IO.Out.KL15  xmono=off  xtype=Double4  xdvaplace=IO_Out  xnstates=0  xfirststate=0  xinitial=0
  Gain : Gain  Gain=10/40
  Gain1 : Gain  Gain=10/60
  ICtrl_AO2 : Terminator
  KL15_SW2 : Subsystem  mask{SignalSelectSwitch=1, SignalConstant=0}
      mask prompts: SignalSelectSwitch "0 FromConstant 1 FromSoftECU"; SignalConstant "ConstantValue"
      mask Display: DispData=get_param(gcbh,'Name');if regexp(DispData,'_');DispData=regexprep(DispData,'_','\\_');end;MaskData=['{\bf\fontsize{12}',DispData,'}'];disp(MaskData, 'texmode','on');
  KL30_SW1 : Subsystem  mask{SignalSelectSwitch=1, SignalConstant=0}
      mask prompts: SignalSelectSwitch "0 FromConstant 1 FromSoftECU"; SignalConstant "ConstantValue"
      mask Display: DispData=get_param(gcbh,'Name');if regexp(DispData,'_');DispData=regexprep(DispData,'_','\\_');end;MaskData=['{\bf\fontsize{12}',DispData,'}'];disp(MaskData, 'texmode','on');
  PwrSupCurrentMor[A] : Gain  Gain=60/10
  PwrSupICtrl[A] : Constant  Value=2
  PwrSupShutDown[0|1] : Constant
  PwrSupUCtrl[V] : Constant  Value=12
  PwrSupVoltageMor[V] : Gain
  Read CM Dict : CarMaker4SL/Read CM Dict  xname=User.IO.Out.KL30  xsync=off
  Read CM Dict1 : CarMaker4SL/Read CM Dict  xname=User.IO.Out.KL15  xsync=off
  Read CM Dict2 : CarMaker4SL/Read CM Dict  xname=User.IO.Out.PwrSupUctrl  xsync=off
  Read CM Dict3 : CarMaker4SL/Read CM Dict  xname=User.IO.Out.PwrSupUctrl_SW  xsync=off
  Saturation : Saturate  UpperLimit=18  LowerLimit=0
  Switch : Switch  Threshold=0.5
  Switch1 : Switch  Criteria=u2 ~= 0
  TB2720_AI1 : Ground
  TB2720_AI2 : Ground
  Terminator : Terminator
  Terminator1 : Terminator
  UCtrl_AO1 : Terminator
  VBAT0_DO1 : Terminator
  Vout0_DO2 : Terminator
  Vout1_DO3 : Terminator
  wires:
  PwrSupICtrl[A]/1 -> Gain1/1
  Gain1/1 -> ICtrl_AO2/1
  PwrSupShutDown[0|1]/1 -> VBAT0_DO1/1, Switch1/2
  Constant/1 -> Switch1/3
  Switch1/1 -> UCtrl_AO1/1
  Gain/1 -> Switch1/1
  TB2720_AI2/1 -> AM_PwrSupVoltageMor/1(In)
  AM_PwrSupVoltageMor/1(Out) -> PwrSupVoltageMor[V]/1
  TB2720_AI1/1 -> AM_PwrSupCurrentMor/1(In)
  AM_PwrSupCurrentMor/1(Out) -> PwrSupCurrentMor[A]/1
  Saturation/1 -> Gain/1
  PwrSupVoltageMor[V]/1 -> Terminator/1  "PwrSupVoltageMor[V]"
  PwrSupCurrentMor[A]/1 -> Terminator1/1  "PwrSupCurrentMor[A]"
  Read CM Dict3/1 -> Switch/2
  Read CM Dict2/1 -> Switch/1
  PwrSupUCtrl[V]/1 -> Switch/3
  Switch/1 -> Saturation/1
  Read CM Dict/1 -> KL30_SW1/1(KL30_SW)
  Read CM Dict1/1 -> KL15_SW2/1(KL30_SW)
  KL30_SW1/1(ToBus_KL30_SW_cause) -> Vout0_DO2/1
  KL15_SW2/1(ToBus_KL30_SW_cause) -> Vout1_DO3/1
